simulink subsystem "HVDCSTATION"  (R2025b)
settings: Solver=VariableStepAuto  StartTime=0.0  StopTime=10.0  RelTol=1e-3
model mask{c=0, vc=0, L=0, VRated=0, SRated=0, t=0, Ts=0}
  mask prompts: c "DC Bus Capacitance (F)"; vc "Capacitor Initial Voltage (V)"; L "Filter Inductance (H)"; VRated "Base Voltage (V)"; SRated "Base Power (VA)"; t "Sensor Time Constant (sec)"; Ts "Sample Time (sec)"
libraries: ee_lib x8, nesl_utility x8, eeGeneralControl x6, fl_lib x4
settings Model: Creator=rajarshd  LastModifiedBy=rajarshd

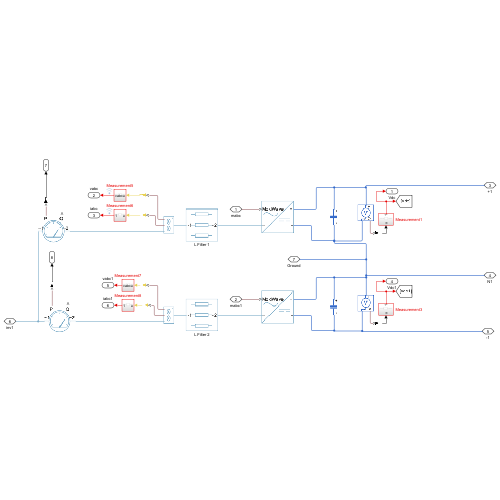
[thumbnail: Simulink's stored preview of the top-level diagram]
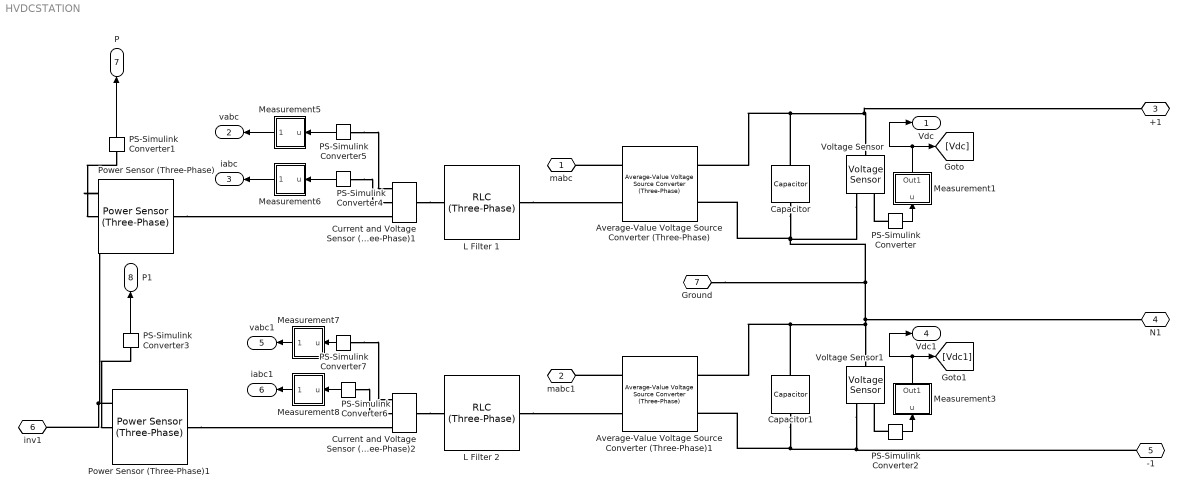
== system HVDCSTATION ==
  Average-Value Voltage Source Converter (Three-Phase) : ee_lib/Semiconductors & Converters/Converters/Average-Value Voltage Source Converter (Three-Phase)  port_option=ee.enum.threePhasePort.composite  frequency_option=ee.enum.converters.frequency.variable  input_option=ee.enum.converters.inputOption.ModWave  FRated=60 Hz  losses_parameterization=ee.enum.converters.losses.fixed  Pfixed=1e-6 W  ks=0.01  kc1=1.7 V  kc2=0.01 Ohm  Ploss_vect=[100, 800, 1870, 3250, 4900] W  Irms_vect=[10, 100, 200, 300, 400] A  Vdc_nom=300 V  thermal_mass=30000 J/K  temperature_specify=off  temperature_priority=High  temperature=298.15 K  temperature_nominal_specify=off  temperature_nominal_value=1  temperature_nominal_unit=K
      settings: InternalSimscapePortConfiguration="{\"Bottom\":[],\"Left\":[{\"id\":\"ModWave\",\"label\":\"ModWave\",\"type\":\"input\"},{\"id\":\"N\",\"label\":\"~\",\"type\":\"foundation.electrical.three_phase\"}],\"Right\":[{\"id\":\"p\",\"label\":\"+\",\"type\":\"foundation.electrical.electrical\"},{\"id\":\"n\",\"label\":\"-\",\"type\":\"foundation.electrical.electrical\"}],\"Top\":[]}"
  Average-Value Voltage Source Converter (Three-Phase)1 : ee_lib/Semiconductors & Converters/Converters/Average-Value Voltage Source Converter (Three-Phase)  port_option=ee.enum.threePhasePort.composite  frequency_option=ee.enum.converters.frequency.variable  input_option=ee.enum.converters.inputOption.ModWave  FRated=60 Hz  losses_parameterization=ee.enum.converters.losses.fixed  Pfixed=1e-6 W  ks=0.01  kc1=1.7 V  kc2=0.01 Ohm  Ploss_vect=[100, 800, 1870, 3250, 4900] W  Irms_vect=[10, 100, 200, 300, 400] A  Vdc_nom=300 V  thermal_mass=30000 J/K  temperature_specify=off  temperature_priority=High  temperature=298.15 K  temperature_nominal_specify=off  temperature_nominal_value=1  temperature_nominal_unit=K
      settings: InternalSimscapePortConfiguration="{\"Bottom\":[],\"Left\":[{\"id\":\"ModWave\",\"label\":\"ModWave\",\"type\":\"input\"},{\"id\":\"N\",\"label\":\"~\",\"type\":\"foundation.electrical.three_phase\"}],\"Right\":[{\"id\":\"p\",\"label\":\"+\",\"type\":\"foundation.electrical.electrical\"},{\"id\":\"n\",\"label\":\"-\",\"type\":\"foundation.electrical.electrical\"}],\"Top\":[]}"
  Capacitor : fl_lib/Electrical/Electrical Elements/Capacitor  c=c F  r=1e-6 Ohm  g=0 1/Ohm  i_specify=off  i_priority=None  i=0 A  i_nominal_specify=off  i_nominal_value=1  i_nominal_unit=A  v_specify=off  v_priority=None  v=6560*.5 V  v_nominal_specify=off  v_nominal_value=1  v_nominal_unit=V  vc_specify=on  vc_priority=High  vc=vc V  vc_nominal_specify=off  vc_nominal_value=1  vc_nominal_unit=V
  Capacitor1 : fl_lib/Electrical/Electrical Elements/Capacitor  c=c F  r=1e-6 Ohm  g=0 1/Ohm  i_specify=off  i_priority=None  i=0 A  i_nominal_specify=off  i_nominal_value=1  i_nominal_unit=A  v_specify=off  v_priority=None  v=6560*.5 V  v_nominal_specify=off  v_nominal_value=1  v_nominal_unit=V  vc_specify=on  vc_priority=High  vc=vc V  vc_nominal_specify=off  vc_nominal_value=1  vc_nominal_unit=V
  Current and Voltage Sensor (Three-Phase)1 : ee_lib/Sensors & Transducers/Current and Voltage Sensor (Three-Phase)  vMeasurementType=ee.enum.vmeasurement.lg  outputUnit=ee.enum.unit.pu  SRated=SRated A*V  VRated=VRated V  I_specify=off  I_priority=None  I=[0, 0, 0] A  I_nominal_specify=off  I_nominal_value=1  I_nominal_unit=A  V_specify=off  V_priority=None  V=[0, 0, 0] V  V_nominal_specify=off  V_nominal_value=1  V_nominal_unit=V
      settings: InternalSimscapePortConfiguration="{\"Bottom\":[],\"Left\":[{\"id\":\"N1\",\"label\":\"~1\",\"type\":\"foundation.electrical.three_phase\"}],\"Right\":[{\"id\":\"V_output\",\"label\":\"V\",\"type\":\"output\"},{\"id\":\"I_output\",\"label\":\"I\",\"type\":\"output\"},{\"id\":\"N2\",\"label\":\"~2\",\"type\":\"foundation.electrical.three_phase\"}],\"Top\":[]}"
  Current and Voltage Sensor (Three-Phase)2 : ee_lib/Sensors & Transducers/Current and Voltage Sensor (Three-Phase)  vMeasurementType=ee.enum.vmeasurement.lg  outputUnit=ee.enum.unit.pu  SRated=SRated A*V  VRated=VRated V  I_specify=off  I_priority=None  I=[0, 0, 0] A  I_nominal_specify=off  I_nominal_value=1  I_nominal_unit=A  V_specify=off  V_priority=None  V=[0, 0, 0] V  V_nominal_specify=off  V_nominal_value=1  V_nominal_unit=V
      settings: InternalSimscapePortConfiguration="{\"Bottom\":[],\"Left\":[{\"id\":\"N1\",\"label\":\"~1\",\"type\":\"foundation.electrical.three_phase\"}],\"Right\":[{\"id\":\"V_output\",\"label\":\"V\",\"type\":\"output\"},{\"id\":\"I_output\",\"label\":\"I\",\"type\":\"output\"},{\"id\":\"N2\",\"label\":\"~2\",\"type\":\"foundation.electrical.three_phase\"}],\"Top\":[]}"
  L Filter 1 : ee_lib/Passive/RLC Assemblies/RLC (Three-Phase)  port_option=ee.enum.threePhasePort.composite  component_structure=ee.enum.rlc.structure.L  R=1e-3 Ohm  L=L H  C=1e-6 F  R_parasitic=0 Ohm  G_parasitic=0 1/Ohm  IL_specify=off  IL_priority=High  IL=[0, 0, 0] A  IL_nominal_specify=off  IL_nominal_value=1  IL_nominal_unit=A  VC_specify=off  VC_priority=High  VC=[0, 0, 0] V  VC_nominal_specify=off  VC_nominal_value=1  VC_nominal_unit=V
      settings: InternalSimscapePortConfiguration="{\"Bottom\":[],\"Left\":[{\"id\":\"N1\",\"label\":\"~1\",\"type\":\"foundation.electrical.three_phase\"}],\"Right\":[{\"id\":\"N2\",\"label\":\"~2\",\"type\":\"foundation.electrical.three_phase\"}],\"Top\":[]}"
  L Filter 2 : ee_lib/Passive/RLC Assemblies/RLC (Three-Phase)  port_option=ee.enum.threePhasePort.composite  component_structure=ee.enum.rlc.structure.L  R=1e-3 Ohm  L=L H  C=1e-6 F  R_parasitic=0 Ohm  G_parasitic=0 1/Ohm  IL_specify=off  IL_priority=High  IL=[0, 0, 0] A  IL_nominal_specify=off  IL_nominal_value=1  IL_nominal_unit=A  VC_specify=off  VC_priority=High  VC=[0, 0, 0] V  VC_nominal_specify=off  VC_nominal_value=1  VC_nominal_unit=V
      settings: InternalSimscapePortConfiguration="{\"Bottom\":[],\"Left\":[{\"id\":\"N1\",\"label\":\"~1\",\"type\":\"foundation.electrical.three_phase\"}],\"Right\":[{\"id\":\"N2\",\"label\":\"~2\",\"type\":\"foundation.electrical.three_phase\"}],\"Top\":[]}"
  Measurement1 : Subsystem
  Measurement3 : Subsystem
  Measurement5 : Subsystem
  Measurement6 : Subsystem
  Measurement7 : Subsystem
  Measurement8 : Subsystem
  PS-Simulink Converter{,1..7} (8 alike) : nesl_utility/PS-Simulink Converter  PhysicalDomain=network_engine_domain  SubClassName=ps_output  LeftPortType=input  RightPortType=output  PseudoPeriodic=off  Frequencies=[]  VectorFormat=inherit  Unit=inherit  AffineConversion=off
  Power Sensor (Three-Phase) : ee_lib/Sensors & Transducers/Power Sensor (Three-Phase)  load_type=ee.enum.passive.type_balanced.balanced  f0=60 Hz
      settings: InternalSimscapePortConfiguration="{\"Bottom\":[],\"Left\":[{\"id\":\"N1\",\"label\":\"~1\",\"type\":\"foundation.electrical.three_phase\"}],\"Right\":[{\"id\":\"N2\",\"label\":\"~2\",\"type\":\"foundation.electrical.three_phase\"}],\"Top\":[{\"id\":\"Pm\",\"label\":\"P\",\"type\":\"output\"},{\"id\":\"Qm\",\"label\":\"Q\",\"type\":\"output\"}]}"
  Power Sensor (Three-Phase)1 : ee_lib/Sensors & Transducers/Power Sensor (Three-Phase)  load_type=ee.enum.passive.type_balanced.balanced  f0=60 Hz
      settings: InternalSimscapePortConfiguration="{\"Bottom\":[],\"Left\":[{\"id\":\"N1\",\"label\":\"~1\",\"type\":\"foundation.electrical.three_phase\"}],\"Right\":[{\"id\":\"N2\",\"label\":\"~2\",\"type\":\"foundation.electrical.three_phase\"}],\"Top\":[{\"id\":\"Pm\",\"label\":\"P\",\"type\":\"output\"},{\"id\":\"Qm\",\"label\":\"Q\",\"type\":\"output\"}]}"
  Voltage Sensor : fl_lib/Electrical/Electrical Sensors/Voltage Sensor
  Voltage Sensor1 : fl_lib/Electrical/Electrical Sensors/Voltage Sensor
  mabc : PMIOPort  Side=Left
  mabc1 : PMIOPort  Port=2  Side=Left
  +1 : PMIOPort  Port=3  Side=Left
  N1 : PMIOPort  Port=4  Side=Left
  -1 : PMIOPort  Port=5  Side=Left
  inv1 : PMIOPort  Port=6  Side=Right
  Ground : PMIOPort  Port=7  Side=Left
  Vdc : Outport
  vabc : Outport  Port=2
  iabc : Outport  Port=3
  Vdc1 : Outport  Port=4
  vabc1 : Outport  Port=5
  iabc1 : Outport  Port=6
  P : Outport  Port=7
  P1 : Outport  Port=8
  wires:
  PS-Simulink Converter/1 -> Measurement1/1(u)
  PS-Simulink Converter2/1 -> Measurement3/1(u)
  Measurement3/1(Out1) -> [Vdc1], Vdc1/1
  PS-Simulink Converter6/1 -> Measurement8/1(u)
  PS-Simulink Converter4/1 -> Measurement6/1(u)
  Measurement8/1(Out1) -> iabc1/1
  Measurement1/1(Out1) -> [Vdc], Vdc/1
  PS-Simulink Converter5/1 -> Measurement5/1(u)
  Measurement6/1(Out1) -> iabc/1
  Measurement7/1(vabc) -> vabc1/1
  Measurement5/1(vabc) -> vabc/1
  PS-Simulink Converter7/1 -> Measurement7/1(u)
  PS-Simulink Converter1/1 -> P/1
  PS-Simulink Converter3/1 -> P1/1
  connections:
  Average-Value Voltage Source Converter (Three-Phase)1/RConn1 -- Capacitor/RConn1 -- Average-Value Voltage Source Converter (Three-Phase)/RConn2 -- Voltage Sensor/RConn2 -- Ground/RConn1 -- N1/RConn1 -- Voltage Sensor1/LConn1 -- Capacitor1/LConn1
  Capacitor/LConn1 -- +1/RConn1 -- Voltage Sensor/LConn1 -- Average-Value Voltage Source Converter (Three-Phase)/RConn1
  Average-Value Voltage Source Converter (Three-Phase)1/RConn2 -- -1/RConn1 -- Voltage Sensor1/RConn2 -- Capacitor1/RConn1
  Power Sensor (Three-Phase)/LConn1 -- Power Sensor (Three-Phase)1/LConn1 -- inv1/RConn1
  L Filter 1/RConn1 -- Average-Value Voltage Source Converter (Three-Phase)/LConn2
  Current and Voltage Sensor (Three-Phase)2/LConn1 -- L Filter 2/LConn1
  Average-Value Voltage Source Converter (Three-Phase)1/LConn1 -- mabc1/RConn1
  PS-Simulink Converter7/LConn1 -- Current and Voltage Sensor (Three-Phase)2/RConn1
  Average-Value Voltage Source Converter (Three-Phase)/LConn1 -- mabc/RConn1
  PS-Simulink Converter6/LConn1 -- Current and Voltage Sensor (Three-Phase)2/RConn2
  Current and Voltage Sensor (Three-Phase)1/LConn1 -- L Filter 1/LConn1
  PS-Simulink Converter2/LConn1 -- Voltage Sensor1/RConn1
  PS-Simulink Converter4/LConn1 -- Current and Voltage Sensor (Three-Phase)1/RConn2
  L Filter 2/RConn1 -- Average-Value Voltage Source Converter (Three-Phase)1/LConn2
  PS-Simulink Converter/LConn1 -- Voltage Sensor/RConn1
  PS-Simulink Converter5/LConn1 -- Current and Voltage Sensor (Three-Phase)1/RConn1
  Power Sensor (Three-Phase)/RConn1 -- Current and Voltage Sensor (Three-Phase)1/RConn3
  Power Sensor (Three-Phase)1/RConn1 -- Current and Voltage Sensor (Three-Phase)2/RConn3
  PS-Simulink Converter1/LConn1 -- Power Sensor (Three-Phase)/LConn2
  PS-Simulink Converter3/LConn1 -- Power Sensor (Three-Phase)1/LConn2

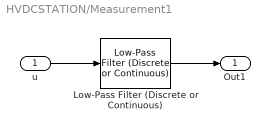
== system HVDCSTATION/Measurement1 ==
  u : Inport
  Low-Pass Filter (Discrete or Continuous) : eeGeneralControl/Low-Pass Filter (Discrete or Continuous)  K=1  T=t  B=inf  A=-inf  init_option=Inherited from block input  x0=0  Ts=-1
  Out1 : Outport
  wires:
  Low-Pass Filter (Discrete or Continuous)/1 -> Out1/1
  u/1 -> Low-Pass Filter (Discrete or Continuous)/1

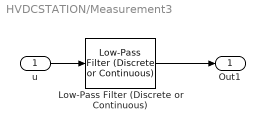
== system HVDCSTATION/Measurement3 ==
  u : Inport
  Low-Pass Filter (Discrete or Continuous) : eeGeneralControl/Low-Pass Filter (Discrete or Continuous)  K=1  T=t  B=inf  A=-inf  init_option=Inherited from block input  x0=0  Ts=-1
  Out1 : Outport
  wires:
  Low-Pass Filter (Discrete or Continuous)/1 -> Out1/1
  u/1 -> Low-Pass Filter (Discrete or Continuous)/1

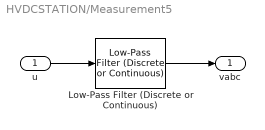
== system HVDCSTATION/Measurement5 ==
  u : Inport
  Low-Pass Filter (Discrete or Continuous) : eeGeneralControl/Low-Pass Filter (Discrete or Continuous)  K=1  T=t  B=inf  A=-inf  init_option=Inherited from block input  x0=0  Ts=-1
  vabc : Outport
  wires:
  Low-Pass Filter (Discrete or Continuous)/1 -> vabc/1
  u/1 -> Low-Pass Filter (Discrete or Continuous)/1

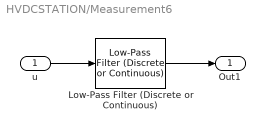
== system HVDCSTATION/Measurement6 ==
  u : Inport
  Low-Pass Filter (Discrete or Continuous) : eeGeneralControl/Low-Pass Filter (Discrete or Continuous)  K=1  T=t  B=inf  A=-inf  init_option=Inherited from block input  x0=0  Ts=-1
  Out1 : Outport
  wires:
  Low-Pass Filter (Discrete or Continuous)/1 -> Out1/1
  u/1 -> Low-Pass Filter (Discrete or Continuous)/1

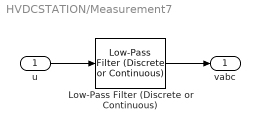
== system HVDCSTATION/Measurement7 ==
  u : Inport
  Low-Pass Filter (Discrete or Continuous) : eeGeneralControl/Low-Pass Filter (Discrete or Continuous)  K=1  T=t  B=inf  A=-inf  init_option=Inherited from block input  x0=0  Ts=-1
  vabc : Outport
  wires:
  Low-Pass Filter (Discrete or Continuous)/1 -> vabc/1
  u/1 -> Low-Pass Filter (Discrete or Continuous)/1

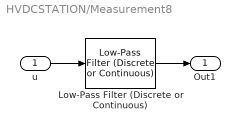
== system HVDCSTATION/Measurement8 ==
  u : Inport
  Low-Pass Filter (Discrete or Continuous) : eeGeneralControl/Low-Pass Filter (Discrete or Continuous)  K=1  T=t  B=inf  A=-inf  init_option=Inherited from block input  x0=0  Ts=-1
  Out1 : Outport
  wires:
  Low-Pass Filter (Discrete or Continuous)/1 -> Out1/1
  u/1 -> Low-Pass Filter (Discrete or Continuous)/1
